simulink model "sim_orbit_min"  (R2025b)
settings: Solver=FixedStepAuto  StartTime=0.0  StopTime=1000  FixedStep=1  RelTol=1e-3
InitFcn:
  | INIT_parametros;
values from neighbouring files (symbols this model uses):
  Cbar = [0	0	0	0 ... (first row only)    [INIT_parametros.m]
  CI_angular = [1;0;0;0;0;0;0]    [INIT_parametros.m]
  CI_lineal = [posicion_inicial;velocidad_inicial]    [INIT_parametros.m]
  GM = 3.986004418e14    (= 398600441800000)    [INIT_parametros.m]    (also in TEST_aerospace_toolbox.m = mu)
  I = [100 0 0 ... (first row only)    [INIT_parametros.m]
  K = [1.000000000000000	0	0	0 ... (first row only)    [INIT_parametros.m]
  m = 1000    [INIT_parametros.m]    (also in TEST_aerospace_toolbox.m = nm_list(ii,2))
  Sbar = [0	0	0	0 ... (first row only)    [INIT_parametros.m]
settings Model: Creator=Allan  LastModifiedBy=Allan
settings OptimizationCC: BlockReduction=off
settings DebuggingCC: AlgebraicLoopMsg=none

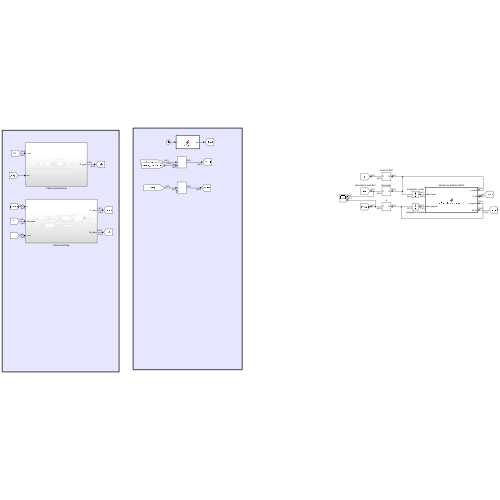
[thumbnail: Simulink's stored preview of the top-level diagram]
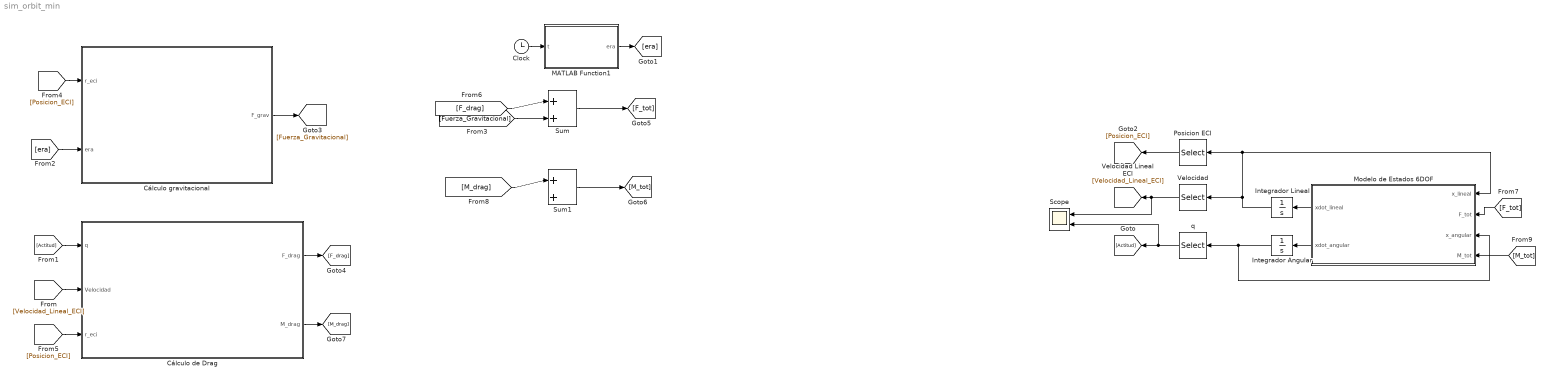
== system sim_orbit_min ==
  Clock : Clock
  Cálculo de Drag : Subsystem
  Cálculo gravitacional : Subsystem
  Integrador Angular : Integrator  InitialCondition=CI_angular
  Integrador Lineal : Integrator  InitialCondition=CI_lineal
  MATLAB Function1 : MATLAB Function  Priority=2  TreatAsAtomicUnit=on
  Modelo de Estados 6DOF : MATLAB Function  TreatAsAtomicUnit=on
  Posicion ECI : Selector  InputPortWidth=6  IndexOptions=Index vector (dialog)  Indices=[1 2 3]  OutputSizes=1  RuntimeRangeChecks=on
  Scope : Scope  NumInputPorts=2
  Sum : Sum  Inputs=|++
  Sum1 : Sum  Inputs=|++
  "Velocidad " : Selector  InputPortWidth=6  IndexOptions=Index vector (dialog)  Indices=[4 5 6]  OutputSizes=1  RuntimeRangeChecks=on
  q : Selector  InputPortWidth=7  IndexOptions=Index vector (dialog)  Indices=[1 2 3 4]  OutputSizes=1  RuntimeRangeChecks=on
  wires:
  Clock/1 -> MATLAB Function1/1(t)
  Integrador Lineal/1 -> Posicion ECI/1, Modelo de Estados 6DOF/1(x_lineal), "Velocidad "/1
  "Velocidad "/1 -> Scope/1, [Velocidad_Lineal_ECI]
  Modelo de Estados 6DOF/1(xdot_lineal) -> Integrador Lineal/1
  Integrador Angular/1 -> q/1, Modelo de Estados 6DOF/3(x_angular)
  [M_tot] -> Modelo de Estados 6DOF/4(M_tot)
  q/1 -> Scope/2, [Actitud]
  [Actitud] -> Cálculo de Drag/1(q)
  [Velocidad_Lineal_ECI] -> Cálculo de Drag/2(Velocidad)
  MATLAB Function1/1(era) -> [era]
  Posicion ECI/1 -> [Posicion_ECI]
  [Posicion_ECI] -> Cálculo de Drag/3(r_eci)
  [era] -> Cálculo gravitacional/2(era)
  [Posicion_ECI] -> Cálculo gravitacional/1(r_eci)
  Cálculo gravitacional/1(F_grav) -> [Fuerza_Gravitacional]
  [F_tot] -> Modelo de Estados 6DOF/2(F_tot)
  Modelo de Estados 6DOF/2(xdot_angular) -> Integrador Angular/1
  Cálculo de Drag/1(F_drag) -> [F_drag]
  [F_drag] -> Sum/1
  Sum/1 -> [F_tot]
  [Fuerza_Gravitacional] -> Sum/2
  Sum1/1 -> [M_tot]
  [M_drag] -> Sum1/1
  Cálculo de Drag/2(M_drag) -> [M_drag]

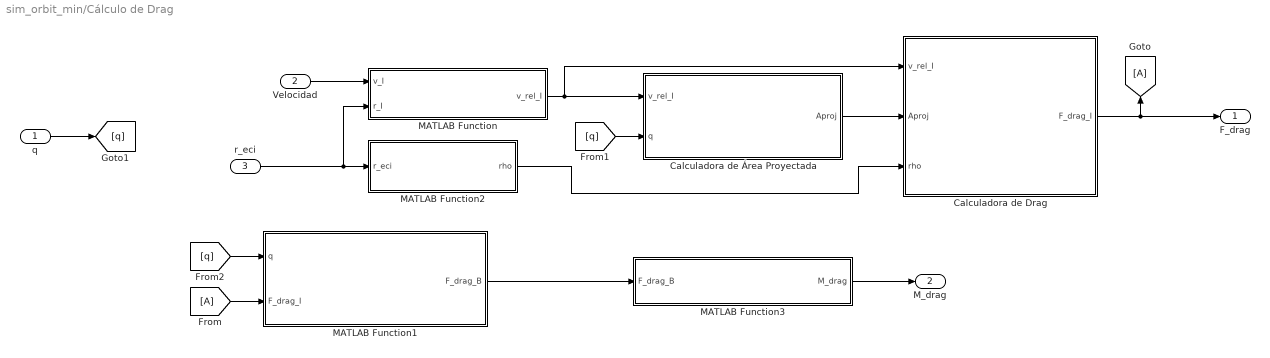
== system sim_orbit_min/Cálculo de Drag ==
  q : Inport
  Velocidad : Inport  Port=2
  r_eci : Inport  Port=3
  Calculadora de Drag : MATLAB Function  TreatAsAtomicUnit=on
  Calculadora de Área Proyectada : MATLAB Function  TreatAsAtomicUnit=on
  From : From
  Goto : Goto
  MATLAB Function : MATLAB Function  TreatAsAtomicUnit=on
  MATLAB Function1 : MATLAB Function  TreatAsAtomicUnit=on
  MATLAB Function2 : MATLAB Function  TreatAsAtomicUnit=on
  MATLAB Function3 : MATLAB Function  TreatAsAtomicUnit=on
  F_drag : Outport
  M_drag : Outport  Port=2  VectorParamsAs1DForOutWhenUnconnected=off
  wires:
  r_eci/1 -> MATLAB Function2/1(r_eci), MATLAB Function/2(r_I)
  MATLAB Function2/1(rho) -> Calculadora de Drag/3(rho)
  Velocidad/1 -> MATLAB Function/1(v_I)
  Calculadora de Drag/1(F_drag_I) -> F_drag/1, Goto/1
  MATLAB Function/1(v_rel_I) -> Calculadora de Drag/1(v_rel_I), Calculadora de Área Proyectada/1(v_rel_I)
  q/1 -> [q]
  [q] -> Calculadora de Área Proyectada/2(q)
  From/1 -> MATLAB Function1/2(F_drag_I)
  [q] -> MATLAB Function1/1(q)
  MATLAB Function1/1(F_drag_B) -> MATLAB Function3/1(F_drag_B)
  MATLAB Function3/1(M_drag) -> M_drag/1
  Calculadora de Área Proyectada/1(Aproj) -> Calculadora de Drag/2(Aproj)

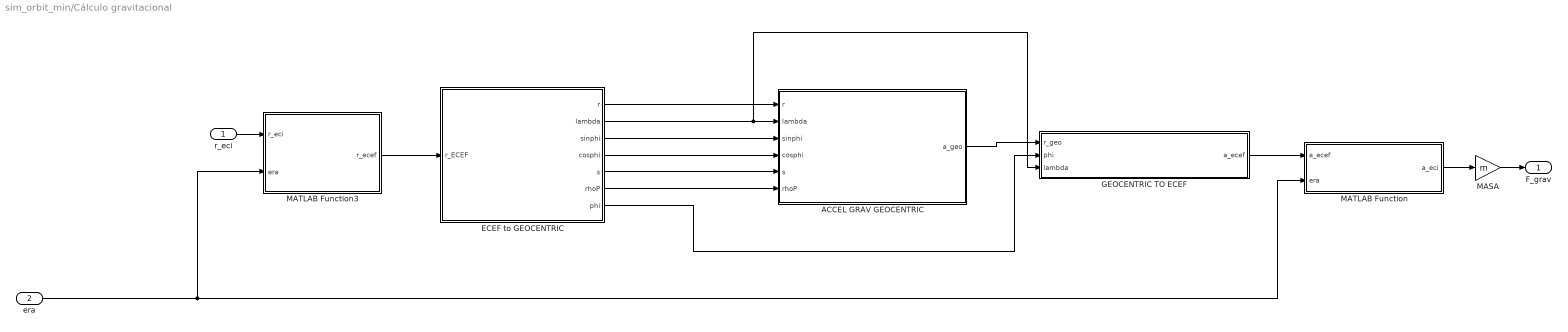
== system sim_orbit_min/Cálculo gravitacional ==
  r_eci : Inport
  era : Inport  Port=2
  ACCEL GRAV GEOCENTRIC : MATLAB Function  TreatAsAtomicUnit=on
  ECEF to GEOCENTRIC : MATLAB Function  TreatAsAtomicUnit=on
  GEOCENTRIC TO ECEF : MATLAB Function  TreatAsAtomicUnit=on
  MASA : Gain  Gain=m
  MATLAB Function : MATLAB Function  TreatAsAtomicUnit=on
  MATLAB Function3 : MATLAB Function  Priority=4  TreatAsAtomicUnit=on
  F_grav : Outport  VectorParamsAs1DForOutWhenUnconnected=off
  wires:
  ACCEL GRAV GEOCENTRIC/1(a_geo) -> GEOCENTRIC TO ECEF/1(r_geo)
  MATLAB Function3/1(r_ecef) -> ECEF to GEOCENTRIC/1(r_ECEF)
  ECEF to GEOCENTRIC/2(lambda) -> GEOCENTRIC TO ECEF/3(lambda), ACCEL GRAV GEOCENTRIC/2(lambda)
  ECEF to GEOCENTRIC/1(r) -> ACCEL GRAV GEOCENTRIC/1(r)
  ECEF to GEOCENTRIC/3(sinphi) -> ACCEL GRAV GEOCENTRIC/3(sinphi)
  ECEF to GEOCENTRIC/4(cosphi) -> ACCEL GRAV GEOCENTRIC/4(cosphi)
  ECEF to GEOCENTRIC/5(s) -> ACCEL GRAV GEOCENTRIC/5(s)
  ECEF to GEOCENTRIC/6(rhoP) -> ACCEL GRAV GEOCENTRIC/6(rhoP)
  GEOCENTRIC TO ECEF/1(a_ecef) -> MATLAB Function/1(a_ecef)
  ECEF to GEOCENTRIC/7(phi) -> GEOCENTRIC TO ECEF/2(phi)
  era/1 -> MATLAB Function3/2(era), MATLAB Function/2(era)
  MATLAB Function/1(a_eci) -> MASA/1
  MASA/1 -> F_grav/1
  r_eci/1 -> MATLAB Function3/1(r_eci)

== matlab function sim_orbit_min/Cálculo de Drag/Calculadora de Drag ==
  data: v_rel_I input; Aproj input; rho input; F_drag_I output; CD parameter
function F_drag_I = MD_drag(v_rel_I, Aproj, rho, CD)
 F_drag_I = MD_drag(v_rel_I,Aproj, rho,CD);
end

== matlab function sim_orbit_min/Cálculo de Drag/Calculadora de Área Proyectada ==
  data: v_rel_I input; q input; Aproj output; A_transversal parameter
function Aproj = MT_area_proyectada(v_rel_I, q, A_transversal)
 Aproj = MT_area_proyectada(v_rel_I, q, A_transversal);
end

== matlab function sim_orbit_min/Cálculo gravitacional/MATLAB Function ==
  data: a_eci output; a_ecef input; era input
function a_eci = MT_ECEF2ECI(a_ecef, era)
    a_eci = MT_ECEF2ECI(a_ecef, era);
end

== matlab function sim_orbit_min/Cálculo de Drag/MATLAB Function1 ==
  data: q input; F_drag_B output; F_drag_I input
function  F_drag_B= MT_INERTIAL2BODY(q,F_drag_I)
  F_drag_B= MT_INERTIAL2BODY(q,F_drag_I);
end

== matlab function sim_orbit_min/Cálculo de Drag/MATLAB Function3 ==
  data: F_drag_B input; M_drag output; CP parameter
function M_drag = MD_momento_drag(F_drag_B, CP)
 M_drag = MD_momento_drag(F_drag_B, CP);
end

== matlab function sim_orbit_min/MATLAB Function1 ==
  data: t input; era output
function era = MD_era(t)
era = MD_era(t);
end

== matlab function sim_orbit_min/Cálculo de Drag/MATLAB Function ==
  data: v_I input; r_I input; v_rel_I output
function v_rel_I = MD_velocidad_relativa(v_I,r_I)
v_rel_I = MD_velocidad_relativa(v_I,r_I);
end

== matlab function sim_orbit_min/Cálculo gravitacional/ACCEL GRAV GEOCENTRIC ==
  data: r input; lambda input; sinphi input; cosphi input; s input; rhoP input; a_geo output; Cbar parameter; Sbar parameter; K parameter; GM parameter
function a_geo = MD_aceleracion_geopotencial(r, lambda, sinphi, cosphi, s, rhoP, Cbar, Sbar, K, GM)
     a_geo = MD_aceleracion_geopotencial(r, lambda, sinphi, cosphi, s, rhoP, Cbar, Sbar, K, GM);
end

== matlab function sim_orbit_min/Cálculo gravitacional/MATLAB Function3 ==
  data: r_eci input; r_ecef output; era input
function r_ecef = MT_ECI2ECEF(r_eci, era)
 r_ecef = MT_ECI2ECEF(r_eci, era);
end

== matlab function sim_orbit_min/Modelo de Estados 6DOF ==
  data: x_lineal input; xdot_lineal output; F_tot input; x_angular input; M_tot input; xdot_angular output; m parameter; I parameter
%% Modelo de estados para un cuerpo rigido con x_lineal = [r(3x1);v(3x1)] y a_angular = [q(4x1);omega(3x1)]
function [xdot_lineal, xdot_angular] = MD_modelo_de_estados(x_lineal,F_tot,x_angular,M_tot,m, I)
    [xdot_lineal, xdot_angular] = MD_modelo_de_estados(x_lineal,F_tot,x_angular,M_tot,m,I);
end

== matlab function sim_orbit_min/Cálculo gravitacional/ECEF to GEOCENTRIC ==
  data: r output; r_ECEF input; lambda output; sinphi output; cosphi output; s output; rhoP output; phi output
function [r, lambda, sinphi, cosphi, s, rhoP,phi] = MT_ECEF2GEOCENTRIC(r_ECEF)
    [r, lambda, sinphi, cosphi, s, rhoP,phi] = MT_ECEF2GEOCENTRIC(r_ECEF);
end

== matlab function sim_orbit_min/Cálculo gravitacional/GEOCENTRIC TO ECEF ==
  data: r_geo input; a_ecef output; phi input; lambda input
function a_ecef = MT_GEOCENTRIC2ECEF(r_geo, phi, lambda)
    a_ecef = MT_GEOCENTRIC2ECEF(r_geo, phi, lambda);
end

== matlab function sim_orbit_min/Cálculo de Drag/MATLAB Function2 ==
  data: r_eci input; rho output
function rho = MD_densidad(r_eci)
rho = MD_densidad(r_eci);
end
